simulink model "Sistema_Fase_Nao_Minima"  (Simulink 7.7)
settings: Solver=ode45  StartTime=0.0  StopTime=20  MaxStep=0.001  RelTol=1e-3
settings Model: Creator=deniseehector  LastModifiedBy=hector
settings OptimizationCC: InitFltsAndDblsToZero=on
settings DebuggingCC: StrictBusMsg=Warning

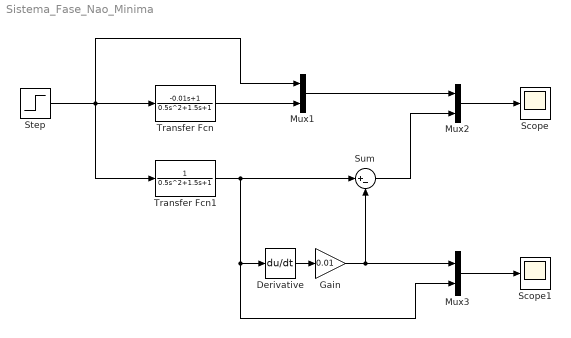
== system Sistema_Fase_Nao_Minima ==
  Derivative : Derivative
  Gain : Gain  Gain=0.01
  Mux1 : Mux  Inputs=2
  Mux2 : Mux  Inputs=2
  Mux3 : Mux  Inputs=2
  Scope : Scope
  Scope1 : Scope
      settings: SaveName=ScopeData2
  Step : Step  SampleTime=0
  Sum : Sum  Inputs=|+-
  Transfer Fcn : TransferFcn  Numerator=[-0.01 1]  Denominator=[0.5 1.5 1]
  Transfer Fcn1 : TransferFcn  Denominator=[0.5 1.5 1]
  wires:
  Step/1 -> Mux1/1, Transfer Fcn/1, Transfer Fcn1/1
  Transfer Fcn/1 -> Mux1/2
  Transfer Fcn1/1 -> Sum/1, Mux3/2, Derivative/1
  Derivative/1 -> Gain/1
  Mux2/1 -> Scope/1
  Sum/1 -> Mux2/2
  Mux1/1 -> Mux2/1
  Mux3/1 -> Scope1/1
  Gain/1 -> Sum/2, Mux3/1
